simulink model "raspberrypi_multicore_simple_tasks_mapped"  (R2021a)
settings: Solver=FixedStepAuto  StartTime=0.0  StopTime=10.0  RelTol=1e-3  EnableMultiTasking=on
undefined symbols (not defined in the file): Green, led0
libraries: simulink x1, raspberrypiBasiclib x1
settings Model: ExplicitPartitioning=on  Creator=The MathWorks, Inc.  LastModifiedBy=The MathWorks, Inc.
settings SolverCC: ConcurrentTasks=on  AlgebraicLoopSolver=TrustRegion  PositivePriorityOrder=on  AutoInsertRateTranBlk=on  InsertRTBMode=Never (minimum delay)
settings OptimizationCC: EnhancedBackFolding=on  PassReuseOutputArgsAs=Individual arguments  ZeroExternalMemoryAtStartup=off  ZeroInternalMemoryAtStartup=off  MaxStackSize=64  OptimizeBlockOrder=speed  DifferentSizesBufferReuse=on  OptimizationCustomize=off  EfficientTunableParamExpr=on
settings DebuggingCC: InheritedTsInSrcMsg=none  ParameterTunabilityLossMsg=error  SFMachineParentedDataDiag=warning
settings HardwareCC: ProdBitPerPointer=32  ProdBitPerSizeT=32  ProdBitPerPtrDiffT=32  ProdLargestAtomicInteger=Long  ProdLargestAtomicFloat=Double  ProdWordSize=32  ProdLongLongMode=on  ProdHWDeviceType=ARM Compatible->ARM Cortex
settings RTWCC: SystemTargetFile=ert.tlc  HardwareBoard=Raspberry Pi  TLCOptions="-aInlineSetEventsForThisBaseRateFcn=TLC_FALSE -aSuppressMultiTaskScheduler=TLC_FALSE  -aRateBasedStepFcn=0"  TemplateMakefile=ert_default_tmf  Toolchain=GNU GCC Embedded Linux  BuildConfiguration=Faster Runs
settings CodeAppCC: ForceParamTrailComments=on  IgnoreCustomStorageClasses=off  OperatorAnnotations=on  SimulinkDataObjDesc=on  SFDataObjDesc=on  InsertBlockDesc=on
settings ERTTargetCC: SupportVariableSizeSignals=on

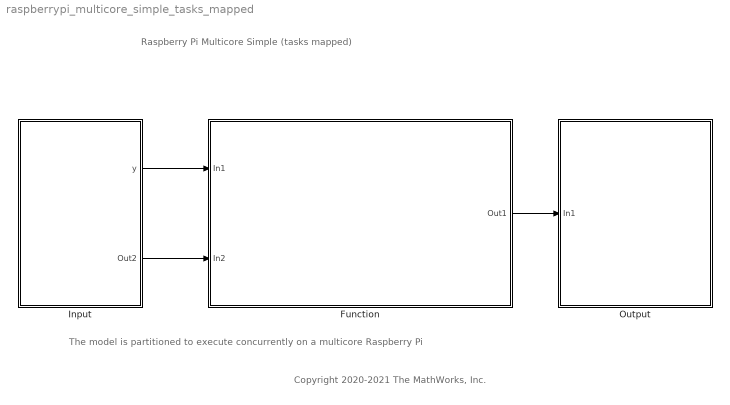
== system raspberrypi_multicore_simple_tasks_mapped ==
  note: The model is partitioned to execute concurrently on a multicore Raspberry Pi
  note: Copyright 2020-2021 The MathWorks, Inc.
  note: Raspberry Pi Multicore Simple (tasks mapped)
  Function : Subsystem  TreatAsAtomicUnit=on
  Input : Subsystem  TreatAsAtomicUnit=on
  Output : Subsystem  TreatAsAtomicUnit=on
  wires:
  Input/1(y) -> Function/1(In1)
  Input/2(Out2) -> Function/2(In2)
  Function/1(Out1) -> Output/1(In1)

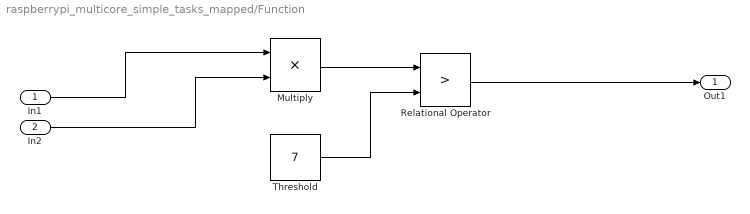
== system raspberrypi_multicore_simple_tasks_mapped/Function ==
  In1 : Inport
  In2 : Inport  Port=2
  Multiply : Product  Inputs=**
  Relational Operator : RelationalOperator  Operator=>  OutDataTypeStr=boolean  RndMeth=Nearest
  "Threshold " : Constant  Value=7  OutDataTypeStr=uint8  SampleTime=-1
  Out1 : Outport
  wires:
  Multiply/1 -> Relational Operator/1
  In2/1 -> Multiply/2
  In1/1 -> Multiply/1
  Relational Operator/1 -> Out1/1
  "Threshold "/1 -> Relational Operator/2

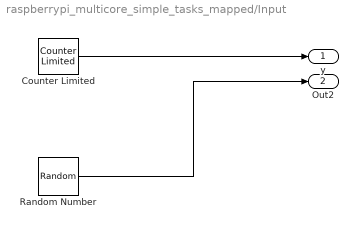
== system raspberrypi_multicore_simple_tasks_mapped/Input ==
  Counter Limited : simulink/Sources/Counter Limited  uplimit=10  tsamp=0.5
  Random Number : RandomNumber
  y : Outport
  Out2 : Outport  Port=2
  wires:
  Counter Limited/1 -> y/1
  Random Number/1 -> Out2/1

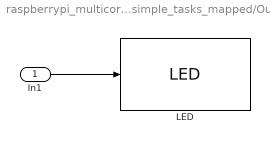
== system raspberrypi_multicore_simple_tasks_mapped/Output ==
  In1 : Inport
  LED : raspberrypiBasiclib/LED  BoardProperty=Model B Rev2  LED_=led0 (Green)
      settings: SourceProductBaseCode=RASPPI
  wires:
  In1/1 -> LED/1
